simulink model "MSD_simul"  (R2022b)
settings: Solver=VariableStepAuto  StartTime=0.0  StopTime=60  RelTol=1e-3
values from neighbouring files (symbols this model uses):
  A = [0 1; -k/m -b/m]    [MSD_parameter.m]
  b = 0.3    [MSD_parameter.m]
  B = [0; 1/m]    [MSD_parameter.m]
  C = [1 0]    [MSD_parameter.m]
  D = 0    [MSD_parameter.m]
  k = 2    [MSD_parameter.m]
  m = 1    [MSD_parameter.m]
undefined symbols (not defined in the file or in its folder): Den, Num
settings Model: Creator=user  LastModifiedBy=user

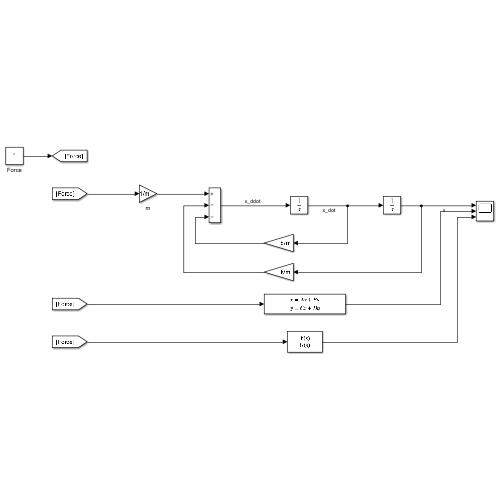
[thumbnail: Simulink's stored preview of the top-level diagram]
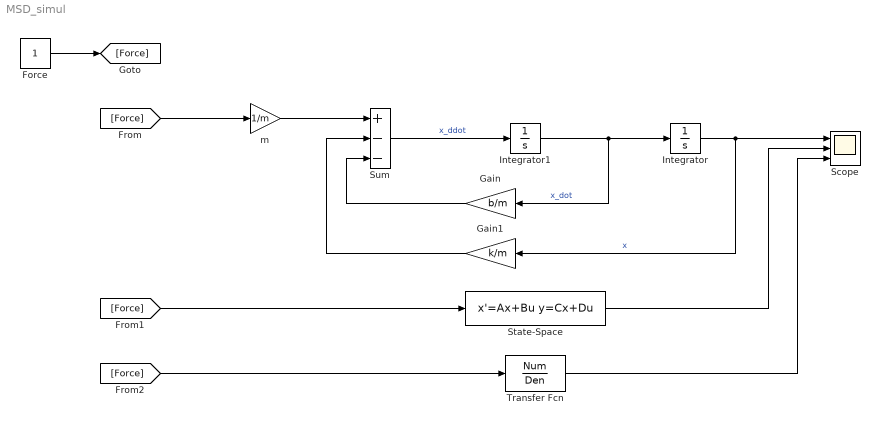
== system MSD_simul ==
  Force : Constant
  Gain : Gain  Gain=b/m
  Gain1 : Gain  Gain=k/m
  Integrator : Integrator
  Integrator1 : Integrator
  Scope : Scope  NumInputPorts=3
  State-Space : StateSpace  A=A  B=B  C=C  D=D  InitialCondition=0
  Sum : Sum  Inputs=+--
  Transfer Fcn : TransferFcn  Numerator=Num  Denominator=Den
  m : Gain  Gain=1/m
  wires:
  Sum/1 -> Integrator1/1  "x_ddot"
  Integrator1/1 -> Gain/1, Integrator/1  "x_dot"
  Integrator/1 -> Scope/1, Gain1/1  "x"
  m/1 -> Sum/1
  Gain/1 -> Sum/3
  Gain1/1 -> Sum/2
  Force/1 -> [Force]
  State-Space/1 -> Scope/2
  [Force] -> m/1
  [Force] -> State-Space/1
  [Force] -> Transfer Fcn/1
  Transfer Fcn/1 -> Scope/3
